simulink library "INT_EBrk_DD"  (R2016b)
settings: Solver=VariableStepAuto  StartTime=0.0  StopTime=10.0  RelTol=1e-3
settings Model: Creator=Administrator  LastModifiedBy=Administrator

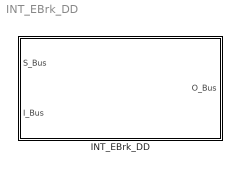
== system INT_EBrk_DD ==
  INT_EBrk_DD : Subsystem

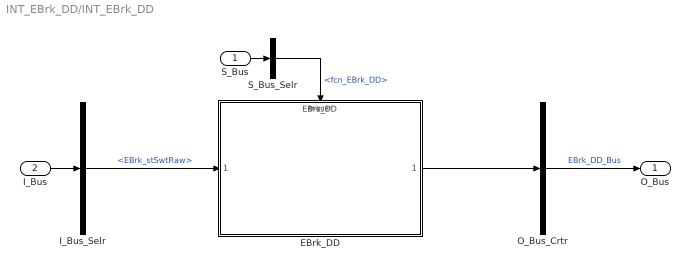
== system INT_EBrk_DD/INT_EBrk_DD ==
  S_Bus : Inport
  I_Bus : Inport  Port=2
  EBrk_DD : ModelReference  ModelNameDialog=EBrk_DD  SimulationMode=Normal  ModelReferenceVersion=1.3  TriggerPortName=function  TriggerPortTriggerType=function-call  TriggerPortStatesWhenEnabling=held
  I_Bus_Selr : BusSelector  OutputSignals=EBrk_stSwtRaw
  O_Bus_Crtr : BusCreator  Inputs=1
  S_Bus_Selr : BusSelector  OutputSignals=fcn_EBrk_DD
  O_Bus : Outport
  wires:
  S_Bus_Selr/1 -> EBrk_DD/Trigger  "<fcn_EBrk_DD>"
  S_Bus/1 -> S_Bus_Selr/1
  I_Bus/1 -> I_Bus_Selr/1
  I_Bus_Selr/1 -> EBrk_DD/1  "<EBrk_stSwtRaw>"
  O_Bus_Crtr/1 -> O_Bus/1  "EBrk_DD_Bus"
  EBrk_DD/1 -> O_Bus_Crtr/1
